simulink model "esercizio3S"  (R2020a)
settings: Solver=VariableStepAuto  StartTime=0.0  StopTime=10.0  RelTol=1e-3
values from neighbouring files (symbols this model uses):
  A = -5    [esempio0.m]    (also in esercizio.m = [-1 -2; 1 -1]; esercizio2.m = [0 2; -10 -12]; esercizio3.m = [0 1; -5 -1]; esercizio4.m = [-7 1; -12 0])
  B = 1    [esempio0.m]    (also in esercizio.m = [0;1]; esercizio2.m = [0;1]; esercizio3.m = [0;1]; esercizio4.m = [0;1])
  C = 1    [esempio0.m]    (also in esercizio.m = [1 0;0 1]; esercizio2.m = [1 0;0 1]; esercizio3.m = [1 0; 0 1]; esercizio4.m = [1 0; 0 1])
  D = 0    [esempio0.m]    (also in esercizio.m = zeros(2,1); esercizio2.m = zeros(2,1); esercizio3.m = zeros(2,1); esercizio4.m = zeros(2,1))
  K = place(A, B, P)    [esempio0.m]    (also in esercizio.m; esercizio2.m; esercizio3.m; esercizio4.m)
  x0 = 0    [esempio0.m]    (also in esercizio2.m = [0;0]; esercizio3.m = [0;0]; esercizio4.m = [0;0])
settings Model: Creator=itama  LastModifiedBy=itama

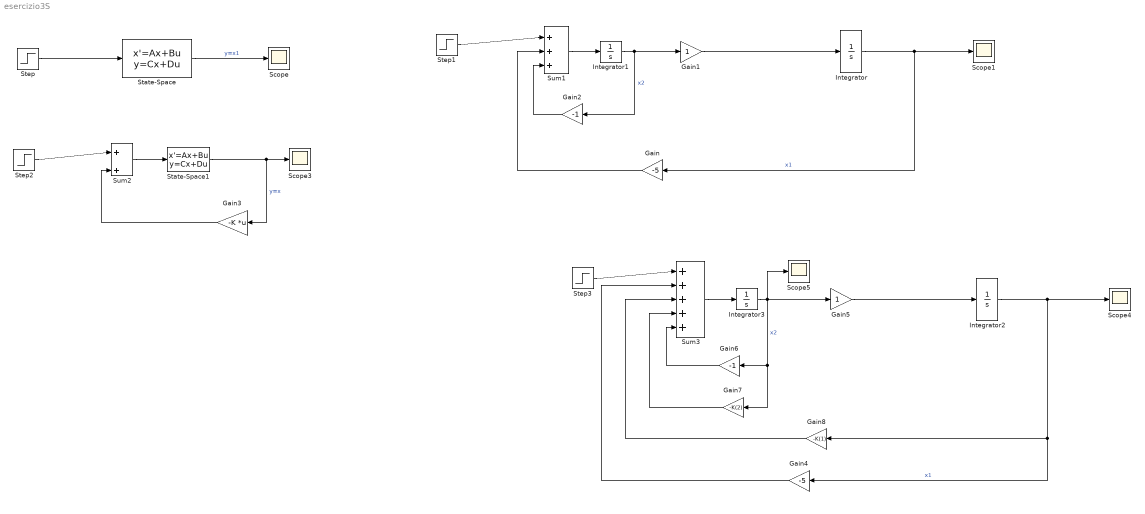
== system esercizio3S ==
  Gain : Gain  Gain=-5
  Gain1 : Gain
  Gain2 : Gain  Gain=-1
  Gain3 : Gain  Gain=-K  Multiplication=Matrix(K*u)
  Gain4 : Gain  Gain=-5
  Gain5 : Gain
  Gain6 : Gain  Gain=-1
  Gain7 : Gain  Gain=-K(2)
  Gain8 : Gain  Gain=-K(1)
  Integrator{,1..3} (4 alike) : Integrator
  Scope{,1,3..5} (5 alike) : Scope
  State-Space : StateSpace  A=A  B=B  C=C  D=D  InitialCondition=x0
  State-Space1 : StateSpace  A=A  B=B  C=C  D=D  InitialCondition=[0;0]
  Step{,1..3} (4 alike) : Step  SampleTime=0
  Sum1 : Sum  Inputs=|+++
  Sum2 : Sum  Inputs=|++
  Sum3 : Sum  Inputs=|+++++
  wires:
  Step/1 -> State-Space/1
  State-Space/1 -> Scope/1  "y=x1"
  Step2/1 -> Sum2/1
  Sum2/1 -> State-Space1/1
  State-Space1/1 -> Gain3/1, Scope3/1  "y=x"
  Gain3/1 -> Sum2/2
  Gain/1 -> Sum1/2
  Integrator/1 -> Gain/1, Scope1/1  "x1"
  Integrator1/1 -> Gain2/1, Gain1/1  "x2"
  Sum1/1 -> Integrator1/1
  Step1/1 -> Sum1/1
  Gain1/1 -> Integrator/1
  Gain2/1 -> Sum1/3
  Gain6/1 -> Sum3/5
  Sum3/1 -> Integrator3/1
  Integrator2/1 -> Gain8/1, Gain4/1, Scope4/1  "x1"
  Gain5/1 -> Integrator2/1
  Integrator3/1 -> Gain7/1, Gain6/1, Gain5/1, Scope5/1  "x2"
  Gain8/1 -> Sum3/3
  Gain4/1 -> Sum3/2
  Step3/1 -> Sum3/1
  Gain7/1 -> Sum3/4
